simulink model "Distribution_v2"  (Simulink 7.9)
settings: Solver=VariableStepDiscrete  StartTime=0.0  StopTime=1000  RelTol=1e-3
libraries: simeventslib x35
(part 6 of 6)

== system Distribution_v2/Customer_9/Commodity_72 ==
  Clock : Clock
  Source : TimeBasedEntityGenerator  Distribution=Exponential  InitialSeed=18340  Mean=Mean  GenerateEntityAtSimulationStart=off
  Timed to Event Signal : TimedToEventSignal
  setAttribute : SetAttribute  AttributeName=Route|Origin|Destination|Start  AttributeFrom=Dialog|Dialog|Dialog|Signal port  AttributeValue="[9  18  22  12]|9|12|1"  AttributeTreatAsVector=0|1|1|1  EvaluatedAttributeValue="{[9  18  22  12];9;12;[]}"
      settings: InputPortMap=u3
  OUT_Commodity : PMIOPort  Port=1  Side=Right
  wires:
  Timed to Event Signal/1 -> setAttribute/1
  Clock/1 -> Timed to Event Signal/1
  connections:
  OUT_Commodity/RConn1 -- setAttribute/RConn1
  Source/RConn1 -- setAttribute/LConn1

== system Distribution_v2/Customer_9/Commodity_73 ==
  Clock : Clock
  Source : TimeBasedEntityGenerator  Distribution=Exponential  InitialSeed=18340  Mean=Mean  GenerateEntityAtSimulationStart=off
  Timed to Event Signal : TimedToEventSignal
  setAttribute : SetAttribute  AttributeName=Route|Origin|Destination|Start  AttributeFrom=Dialog|Dialog|Dialog|Signal port  AttributeValue="[9  18  20  14]|9|14|1"  AttributeTreatAsVector=0|1|1|1  EvaluatedAttributeValue="{[9  18  20  14];9;14;[]}"
      settings: InputPortMap=u3
  OUT_Commodity : PMIOPort  Port=1  Side=Right
  wires:
  Timed to Event Signal/1 -> setAttribute/1
  Clock/1 -> Timed to Event Signal/1
  connections:
  OUT_Commodity/RConn1 -- setAttribute/RConn1
  Source/RConn1 -- setAttribute/LConn1

== system Distribution_v2/Customer_9/Commodity_74 ==
  Clock : Clock
  Source : TimeBasedEntityGenerator  Distribution=Exponential  InitialSeed=18340  Mean=Mean  GenerateEntityAtSimulationStart=off
  Timed to Event Signal : TimedToEventSignal
  setAttribute : SetAttribute  AttributeName=Route|Origin|Destination|Start  AttributeFrom=Dialog|Dialog|Dialog|Signal port  AttributeValue="[9  18  20  15]|9|15|1"  AttributeTreatAsVector=0|1|1|1  EvaluatedAttributeValue="{[9  18  20  15];9;15;[]}"
      settings: InputPortMap=u3
  OUT_Commodity : PMIOPort  Port=1  Side=Right
  wires:
  Timed to Event Signal/1 -> setAttribute/1
  Clock/1 -> Timed to Event Signal/1
  connections:
  OUT_Commodity/RConn1 -- setAttribute/RConn1
  Source/RConn1 -- setAttribute/LConn1

== system Distribution_v2/Depot_18/Resource_Pool ==
  Event-Based Entity Generator : EventBasedEntityGenerator  GenerateEntitiesUpon=Function call from port fcn
  FIFO Queue : FIFOQueue  Capacity=8
  Path Combiner : PathCombiner  NumberInputPorts=2
  Time-Based Function-Call Generator : TimeBasedFunctionCallGenerator  EventGenerationMode=Only at simulation start  NumberOfEventsPerPeriod=Quantity
  Acquire : PMIOPort  Port=1  Side=Left
  Return : PMIOPort  Port=2  Side=Right
  wires:
  Time-Based Function-Call Generator/1 -> Event-Based Entity Generator/1
  connections:
  Acquire/RConn1 -- FIFO Queue/RConn1
  Return/RConn1 -- Path Combiner/LConn2
  Path Combiner/RConn1 -- FIFO Queue/LConn1
  Event-Based Entity Generator/RConn1 -- Path Combiner/LConn1

== system Distribution_v2/Depot_20/Resource_Pool ==
  Event-Based Entity Generator : EventBasedEntityGenerator  GenerateEntitiesUpon=Function call from port fcn
  FIFO Queue : FIFOQueue  Capacity=8
  Path Combiner : PathCombiner  NumberInputPorts=2
  Time-Based Function-Call Generator : TimeBasedFunctionCallGenerator  EventGenerationMode=Only at simulation start  NumberOfEventsPerPeriod=Quantity
  Acquire : PMIOPort  Port=1  Side=Left
  Return : PMIOPort  Port=2  Side=Right
  wires:
  Time-Based Function-Call Generator/1 -> Event-Based Entity Generator/1
  connections:
  Acquire/RConn1 -- FIFO Queue/RConn1
  Return/RConn1 -- Path Combiner/LConn2
  Path Combiner/RConn1 -- FIFO Queue/LConn1
  Event-Based Entity Generator/RConn1 -- Path Combiner/LConn1

== system Distribution_v2/Depot_22/Resource_Pool ==
  Event-Based Entity Generator : EventBasedEntityGenerator  GenerateEntitiesUpon=Function call from port fcn
  FIFO Queue : FIFOQueue  Capacity=8
  Path Combiner : PathCombiner  NumberInputPorts=2
  Time-Based Function-Call Generator : TimeBasedFunctionCallGenerator  EventGenerationMode=Only at simulation start  NumberOfEventsPerPeriod=Quantity
  Acquire : PMIOPort  Port=1  Side=Left
  Return : PMIOPort  Port=2  Side=Right
  wires:
  Time-Based Function-Call Generator/1 -> Event-Based Entity Generator/1
  connections:
  Acquire/RConn1 -- FIFO Queue/RConn1
  Return/RConn1 -- Path Combiner/LConn2
  Path Combiner/RConn1 -- FIFO Queue/LConn1
  Event-Based Entity Generator/RConn1 -- Path Combiner/LConn1

== matlab function Depot_20/Control: Resource Allocation ==
  data: IN_1 input double; OUT_1 output double; IN_2 input double; IN_3 input double; IN_4 input double; IN_5 input double; IN_6 input double; IN_7 input double; IN_8 input double; IN_9 input double; IN_10 input double; IN_11 input double; IN_12 input double; last input double
  events: Release output FUNCTION_CALL_EVENT
function OUT_1 = resource_alloc(IN_1, IN_2, IN_3, IN_4, IN_5, IN_6, IN_7, IN_8, IN_9, IN_10, IN_11, IN_12, last)
%#codegen

OUT_1 = 1;

if last ==0
    last =1;
end

Policy = 'Longest Queue';
Status = zeros(12,3);

if length(IN_12)>1
    Status(12,:) = [IN_12'];
else
    Status = zeros(11,3);
end
if length(IN_11)>1
    Status(11,:) = [IN_11'];
else
    Status = zeros(10,3);
end
if length(IN_10)>1
    Status(10,:) = [IN_10'];
else
    Status = zeros(9,3);
end
if length(IN_9)>1
    Status(9,:) = [IN_9'];
else
    Status = zeros(8,3);
end
if length(IN_8)>1
    Status(8,:) = [IN_8'];
else
    Status = zeros(7,3);
end
if length(IN_7)>1
    Status(7,:) = [IN_7'];
else
    Status = zeros(6,3);
end
if length(IN_6)>1
    Status(6,:) = [IN_6'];
else
    Status = zeros(5,3);
end

if length(IN_5)>1
    Status(5,:) = [IN_5'];
else
    Status = zeros(4,3);
end
if length(IN_4)>1
    Status(4,:) = [IN_4'];
else
    Status = zeros(3,3);
end
if length(IN_3)>1
    Status(3,:) = [IN_3'];
else
    Status = zeros(2,3);
end
if length(IN_2)>1
    Status(2,:) = [IN_2'];
else
    Status = zeros(1,3);
end

Status(1,:) = [IN_1'];

        


if strcmp(Policy, 'Longest Queue') ==1
    Status(last, :) = [NaN, NaN, NaN];
    y = min(Status(:,2));
    x = max(Status(Status(:,2)==y));

    for i = 1:length(Status(:,1))
       if Status(i,1)== x && Status(i,2) == y
           Release;
           OUT_1 = i;
           last = i;
           break;
       end
    end
    
elseif strcmp(Policy, 'Min Queue') ==1
    Status(last, :) = [NaN, NaN, NaN];
    y = min(Status(:,2));
    x = max(Status(Status(:,2)==y));

    for i = 1:length(Status(:,1))
       if Status(i,1)== x && Status(i,2) == y && Status(i,1)>10 && Status(i,2)<2
           Release;
           OUT_1 = i;
           last =i;
           break;
       end
    end
else %Round-Robin
    PortCount = length(Status);
    
    if last == PortCount
        OUT_1 = 1;
        last = last+1;
    else
        OUT_1 = last +1;
        last = last+1;
    end
    Release;
end

== matlab function Depot_18/MATLAB Function ==
  data: route input double; next output double; current input double; lookup input double
function next = routing(route, current, lookup)
%#codegen
next = 1;
for i = 1:length(route)
   if route(i) == current
       next = route(i+1);
   end
   
   for j = 1:length(lookup)
       if lookup(j) == next
           next = j;
       end
   end
end

== matlab function Depot_20/MATLAB Function ==
  data: route input double; next output double; current input double; lookup input double
function next = routing(route, current, lookup)
%#codegen
next = 1;
for i = 1:length(route)
   if route(i) == current
       next = route(i+1);
   end
   
   for j = 1:length(lookup)
       if lookup(j) == next
           next = j;
       end
   end
end

== matlab function Depot_18/Control: Resource Allocation ==
  data: IN_1 input double; OUT_1 output double; IN_2 input double; IN_3 input double; IN_4 input double; IN_5 input double; IN_6 input double; IN_7 input double; IN_8 input double; IN_9 input double; IN_10 input double; IN_11 input double; IN_12 input double; last input double
  events: Release output FUNCTION_CALL_EVENT
function OUT_1 = resource_alloc(IN_1, IN_2, IN_3, IN_4, IN_5, IN_6, IN_7, IN_8, IN_9, IN_10, IN_11, IN_12, last)
%#codegen

OUT_1 = 1;

if last ==0
    last =1;
end

Policy = 'Longest Queue';
Status = zeros(12,3);

if length(IN_12)>1
    Status(12,:) = [IN_12'];
else
    Status = zeros(11,3);
end
if length(IN_11)>1
    Status(11,:) = [IN_11'];
else
    Status = zeros(10,3);
end
if length(IN_10)>1
    Status(10,:) = [IN_10'];
else
    Status = zeros(9,3);
end
if length(IN_9)>1
    Status(9,:) = [IN_9'];
else
    Status = zeros(8,3);
end
if length(IN_8)>1
    Status(8,:) = [IN_8'];
else
    Status = zeros(7,3);
end
if length(IN_7)>1
    Status(7,:) = [IN_7'];
else
    Status = zeros(6,3);
end
if length(IN_6)>1
    Status(6,:) = [IN_6'];
else
    Status = zeros(5,3);
end

if length(IN_5)>1
    Status(5,:) = [IN_5'];
else
    Status = zeros(4,3);
end
if length(IN_4)>1
    Status(4,:) = [IN_4'];
else
    Status = zeros(3,3);
end
if length(IN_3)>1
    Status(3,:) = [IN_3'];
else
    Status = zeros(2,3);
end
if length(IN_2)>1
    Status(2,:) = [IN_2'];
else
    Status = zeros(1,3);
end

Status(1,:) = [IN_1'];

        


if strcmp(Policy, 'Longest Queue') ==1
    Status(last, :) = [NaN, NaN, NaN];
    y = min(Status(:,2));
    x = max(Status(Status(:,2)==y));

    for i = 1:length(Status(:,1))
       if Status(i,1)== x && Status(i,2) == y
           Release;
           OUT_1 = i;
           last = i;
           break;
       end
    end
    
elseif strcmp(Policy, 'Min Queue') ==1
    Status(last, :) = [NaN, NaN, NaN];
    y = min(Status(:,2));
    x = max(Status(Status(:,2)==y));

    for i = 1:length(Status(:,1))
       if Status(i,1)== x && Status(i,2) == y && Status(i,1)>10 && Status(i,2)<2
           Release;
           OUT_1 = i;
           last =i;
           break;
       end
    end
else %Round-Robin
    PortCount = length(Status);
    
    if last == PortCount
        OUT_1 = 1;
        last = last+1;
    else
        OUT_1 = last +1;
        last = last+1;
    end
    Release;
end

== matlab function Depot_22/Control: Resource Allocation ==
  data: IN_1 input double; OUT_1 output double; IN_2 input double; IN_3 input double; IN_4 input double; IN_5 input double; IN_6 input double; IN_7 input double; IN_8 input double; IN_9 input double; IN_10 input double; IN_11 input double; IN_12 input double; last input double
  events: Release output FUNCTION_CALL_EVENT
function OUT_1 = resource_alloc(IN_1, IN_2, IN_3, IN_4, IN_5, IN_6, IN_7, IN_8, IN_9, IN_10, IN_11, IN_12, last)
%#codegen

OUT_1 = 1;

if last ==0
    last =1;
end

Policy = 'Longest Queue';
Status = zeros(12,3);

if length(IN_12)>1
    Status(12,:) = [IN_12'];
else
    Status = zeros(11,3);
end
if length(IN_11)>1
    Status(11,:) = [IN_11'];
else
    Status = zeros(10,3);
end
if length(IN_10)>1
    Status(10,:) = [IN_10'];
else
    Status = zeros(9,3);
end
if length(IN_9)>1
    Status(9,:) = [IN_9'];
else
    Status = zeros(8,3);
end
if length(IN_8)>1
    Status(8,:) = [IN_8'];
else
    Status = zeros(7,3);
end
if length(IN_7)>1
    Status(7,:) = [IN_7'];
else
    Status = zeros(6,3);
end
if length(IN_6)>1
    Status(6,:) = [IN_6'];
else
    Status = zeros(5,3);
end

if length(IN_5)>1
    Status(5,:) = [IN_5'];
else
    Status = zeros(4,3);
end
if length(IN_4)>1
    Status(4,:) = [IN_4'];
else
    Status = zeros(3,3);
end
if length(IN_3)>1
    Status(3,:) = [IN_3'];
else
    Status = zeros(2,3);
end
if length(IN_2)>1
    Status(2,:) = [IN_2'];
else
    Status = zeros(1,3);
end

Status(1,:) = [IN_1'];

        


if strcmp(Policy, 'Longest Queue') ==1
    Status(last, :) = [NaN, NaN, NaN];
    y = min(Status(:,2));
    x = max(Status(Status(:,2)==y));

    for i = 1:length(Status(:,1))
       if Status(i,1)== x && Status(i,2) == y
           Release;
           OUT_1 = i;
           last = i;
           break;
       end
    end
    
elseif strcmp(Policy, 'Min Queue') ==1
    Status(last, :) = [NaN, NaN, NaN];
    y = min(Status(:,2));
    x = max(Status(Status(:,2)==y));

    for i = 1:length(Status(:,1))
       if Status(i,1)== x && Status(i,2) == y && Status(i,1)>10 && Status(i,2)<2
           Release;
           OUT_1 = i;
           last =i;
           break;
       end
    end
else %Round-Robin
    PortCount = length(Status);
    
    if last == PortCount
        OUT_1 = 1;
        last = last+1;
    else
        OUT_1 = last +1;
        last = last+1;
    end
    Release;
end

== matlab function Depot_22/MATLAB Function ==
  data: route input double; next output double; current input double; lookup input double
function next = routing(route, current, lookup)
%#codegen
next = 1;
for i = 1:length(route)
   if route(i) == current
       next = route(i+1);
   end
   
   for j = 1:length(lookup)
       if lookup(j) == next
           next = j;
       end
   end
end

== matlab function Customer_1/MATLAB Function ==
  data: route input double; next output double; current input double; lookup input double
function next = routing(route, current, lookup)
%#codegen
next = 1;
for i = 1:length(route)
   if route(i) == current
       next = route(i+1);
   end
   
   for j = 1:length(lookup)
       if lookup(j) == next
           next = j;
       end
   end
end

== matlab function Customer_2/MATLAB Function ==
  data: route input double; next output double; current input double; lookup input double
function next = routing(route, current, lookup)
%#codegen
next = 1;
for i = 1:length(route)
   if route(i) == current
       next = route(i+1);
   end
   
   for j = 1:length(lookup)
       if lookup(j) == next
           next = j;
       end
   end
end

== matlab function Customer_3/MATLAB Function ==
  data: route input double; next output double; current input double; lookup input double
function next = routing(route, current, lookup)
%#codegen
next = 1;
for i = 1:length(route)
   if route(i) == current
       next = route(i+1);
   end
   
   for j = 1:length(lookup)
       if lookup(j) == next
           next = j;
       end
   end
end

== matlab function Customer_4/MATLAB Function ==
  data: route input double; next output double; current input double; lookup input double
function next = routing(route, current, lookup)
%#codegen
next = 1;
for i = 1:length(route)
   if route(i) == current
       next = route(i+1);
   end
   
   for j = 1:length(lookup)
       if lookup(j) == next
           next = j;
       end
   end
end

== matlab function Customer_5/MATLAB Function ==
  data: route input double; next output double; current input double; lookup input double
function next = routing(route, current, lookup)
%#codegen
next = 1;
for i = 1:length(route)
   if route(i) == current
       next = route(i+1);
   end
   
   for j = 1:length(lookup)
       if lookup(j) == next
           next = j;
       end
   end
end

== matlab function Customer_6/MATLAB Function ==
  data: route input double; next output double; current input double; lookup input double
function next = routing(route, current, lookup)
%#codegen
next = 1;
for i = 1:length(route)
   if route(i) == current
       next = route(i+1);
   end
   
   for j = 1:length(lookup)
       if lookup(j) == next
           next = j;
       end
   end
end

== matlab function Customer_7/MATLAB Function ==
  data: route input double; next output double; current input double; lookup input double
function next = routing(route, current, lookup)
%#codegen
next = 1;
for i = 1:length(route)
   if route(i) == current
       next = route(i+1);
   end
   
   for j = 1:length(lookup)
       if lookup(j) == next
           next = j;
       end
   end
end

== matlab function Customer_8/MATLAB Function ==
  data: route input double; next output double; current input double; lookup input double
function next = routing(route, current, lookup)
%#codegen
next = 1;
for i = 1:length(route)
   if route(i) == current
       next = route(i+1);
   end
   
   for j = 1:length(lookup)
       if lookup(j) == next
           next = j;
       end
   end
end

== matlab function Customer_9/MATLAB Function ==
  data: route input double; next output double; current input double; lookup input double
function next = routing(route, current, lookup)
%#codegen
next = 1;
for i = 1:length(route)
   if route(i) == current
       next = route(i+1);
   end
   
   for j = 1:length(lookup)
       if lookup(j) == next
           next = j;
       end
   end
end

== matlab function Customer_10/MATLAB Function ==
  data: route input double; next output double; current input double; lookup input double
function next = routing(route, current, lookup)
%#codegen
next = 1;
for i = 1:length(route)
   if route(i) == current
       next = route(i+1);
   end
   
   for j = 1:length(lookup)
       if lookup(j) == next
           next = j;
       end
   end
end

== matlab function Customer_11/MATLAB Function ==
  data: route input double; next output double; current input double; lookup input double
function next = routing(route, current, lookup)
%#codegen
next = 1;
for i = 1:length(route)
   if route(i) == current
       next = route(i+1);
   end
   
   for j = 1:length(lookup)
       if lookup(j) == next
           next = j;
       end
   end
end

== matlab function Customer_12/MATLAB Function ==
  data: route input double; next output double; current input double; lookup input double
function next = routing(route, current, lookup)
%#codegen
next = 1;
for i = 1:length(route)
   if route(i) == current
       next = route(i+1);
   end
   
   for j = 1:length(lookup)
       if lookup(j) == next
           next = j;
       end
   end
end

== matlab function Customer_13/MATLAB Function ==
  data: route input double; next output double; current input double; lookup input double
function next = routing(route, current, lookup)
%#codegen
next = 1;
for i = 1:length(route)
   if route(i) == current
       next = route(i+1);
   end
   
   for j = 1:length(lookup)
       if lookup(j) == next
           next = j;
       end
   end
end

== matlab function Customer_14/MATLAB Function ==
  data: route input double; next output double; current input double; lookup input double
function next = routing(route, current, lookup)
%#codegen
next = 1;
for i = 1:length(route)
   if route(i) == current
       next = route(i+1);
   end
   
   for j = 1:length(lookup)
       if lookup(j) == next
           next = j;
       end
   end
end

== matlab function Customer_15/MATLAB Function ==
  data: route input double; next output double; current input double; lookup input double
function next = routing(route, current, lookup)
%#codegen
next = 1;
for i = 1:length(route)
   if route(i) == current
       next = route(i+1);
   end
   
   for j = 1:length(lookup)
       if lookup(j) == next
           next = j;
       end
   end
end
